simulink model "jacobian_inverse"  (R2019b)
settings: Solver=VariableStepAuto  StartTime=0.0  StopTime=4.0  RelTol=1e-3
undefined symbols (not defined in the file or in its folder): DiscIntNeverNeededParam, q0, Tc
settings Model: Creator=rajath  LastModifiedBy=GA

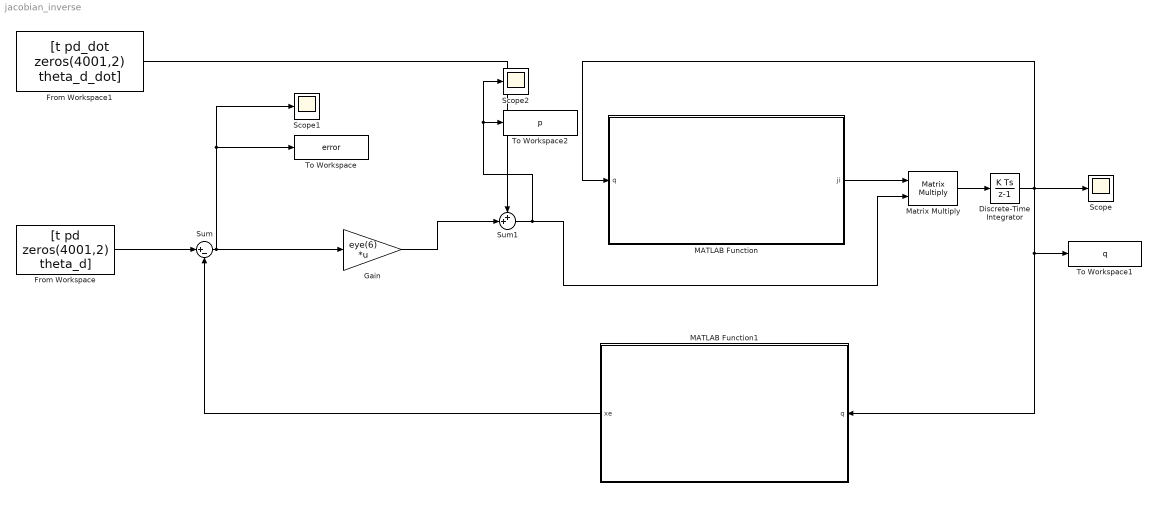
== system jacobian_inverse ==
  Discrete-Time Integrator : DiscreteIntegrator  gainval=1  InitialCondition=q0  SampleTime=Tc  ICPrevOutput=DiscIntNeverNeededParam  ICPrevScaledInput=DiscIntNeverNeededParam
  From Workspace : FromWorkspace  VariableName=[t pd zeros(4001,2) theta_d]  SampleTime=Tc
  From Workspace1 : FromWorkspace  VariableName=[t pd_dot zeros(4001,2) theta_d_dot]  SampleTime=Tc
  Gain : Gain  Gain=eye(6)  Multiplication=Matrix(K*u)
  MATLAB Function : MATLAB Function  TreatAsAtomicUnit=on
  MATLAB Function1 : MATLAB Function  TreatAsAtomicUnit=on
  Matrix Multiply : Product  Multiplication=Matrix(*)
  Scope : Scope
  Scope1 : Scope
  Scope2 : Scope
  Sum : Sum  Inputs=|+-
  Sum1 : Sum  Inputs=++|
  To Workspace : ToWorkspace  VariableName=error  SaveFormat=Timeseries  SampleTime=Tc
  To Workspace1 : ToWorkspace  VariableName=q  SaveFormat=Timeseries  SampleTime=-1
  To Workspace2 : ToWorkspace  VariableName=p  SaveFormat=Timeseries  SampleTime=Tc
  wires:
  From Workspace/1 -> Sum/1
  Sum/1 -> Gain/1, Scope1/1, To Workspace/1
  From Workspace1/1 -> Sum1/1
  Discrete-Time Integrator/1 -> MATLAB Function/1(q), Scope/1, To Workspace1/1, MATLAB Function1/1(q)
  MATLAB Function1/1(xe) -> Sum/2
  MATLAB Function/1(ji) -> Matrix Multiply/1
  Matrix Multiply/1 -> Discrete-Time Integrator/1
  Gain/1 -> Sum1/2
  Sum1/1 -> To Workspace2/1, Scope2/1, Matrix Multiply/2

== matlab function jacobian_inverse/MATLAB Function1 ==
  data: q input; xe output
function xe = non_linear_function(q)
a1 = 0.5;
a2 = 0.5;
d0 = 1;
xe = zeros(6,1);
xe(1,:) = a1*cos(q(1))+a2*cos(q(1)+q(2));
xe(2,:) = a1*sin(q(1))+a2*sin(q(1)+q(2));
xe(3,:) = d0 - q(3);
xe(4,:) = 0;
xe(5,:) = 0;
xe(6,:) = asin(sin(q(1)+q(2)+q(4)));

== matlab function jacobian_inverse/MATLAB Function ==
  data: q input; ji output
function ji = jacobian_inverse(q)
    
a1 = 0.5;
a2 = 0.5;

j = zeros(6,4);
j(1,1) = -a1*sin(q(1))-a2*sin(q(1)+q(2));
j(1,2) = -a2*sin(q(1)+q(2));
j(2,1) = a1*cos(q(1))+a2*cos(q(1)+q(2));
j(2,2) = a2*cos(q(1)+q(2));
j(3,3) = -1;
j(6,1) = 1;
j(6,2) = 1;
j(6,4) = -1;
ji = pinv(j);
